simulink model "SHELL"  (Simulink 10.2)
settings: Solver=VariableStepAuto  StartTime=0.0  StopTime="sim_par.t_end  "  FixedStep=sim_par.dt  MaxStep="sim_par.t_step  "  RelTol="sim_par.rel_solver_tol "  EnableMultiTasking=on
libraries: OBSW x1, RWSW x1
settings Model: Creator=alger  LastModifiedBy=dbell44
settings DataIOCC: LimitDataPoints=on  SignalLoggingSaveFormat=Dataset
settings DebuggingCC: SolverPrmCheckMsg=warning  FcnCallInpInsideContextMsg=error  SignalLabelMismatchMsg=warning  UnconnectedLineMsg=error  RootOutportRequireBusObject=none  StateNameClashWarn=warning  StrictBusMsg=WarnOnBusTreatedAsVector  NonBusSignalsTreatedAsBus=warning
settings GRTTargetCC: CombineOutputUpdateFcns=on  GRTInterface=off

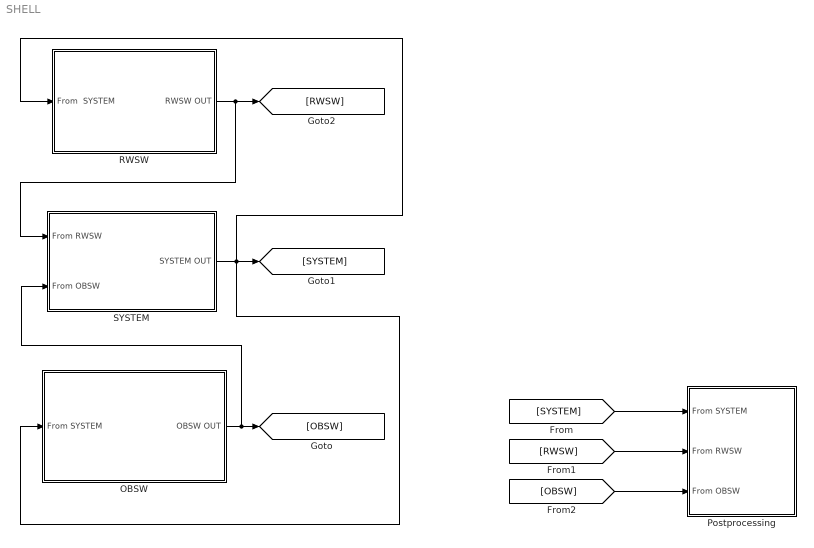
== system SHELL ==
  OBSW : Subsystem
  Postprocessing : Subsystem
  RWSW : Subsystem
  SYSTEM : Subsystem
  wires:
  OBSW/1(OBSW OUT) -> SYSTEM/2(From OBSW), [OBSW]
  [SYSTEM] -> Postprocessing/1(From SYSTEM)
  [RWSW] -> Postprocessing/2(From RWSW)
  [OBSW] -> Postprocessing/3("From OBSW ")
  RWSW/1(RWSW OUT) -> [RWSW], SYSTEM/1(From RWSW)
  SYSTEM/1("SYSTEM OUT ") -> [SYSTEM], OBSW/1(From SYSTEM), RWSW/1(From  SYSTEM)

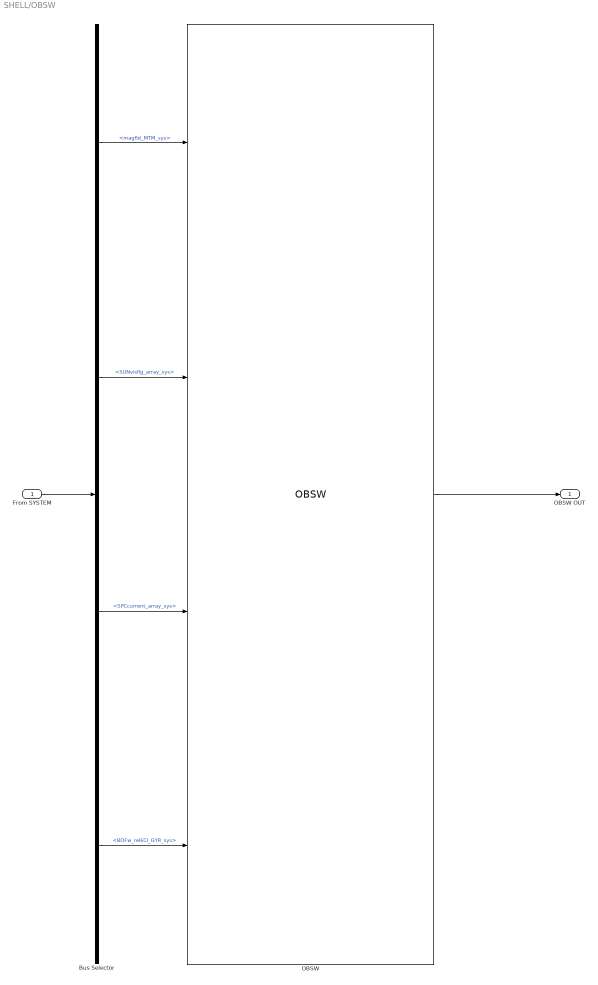
== system SHELL/OBSW ==
  From SYSTEM : Inport
  Bus Selector : BusSelector  OutputSignals=SYSSEN.magfld_MTM_sys,SYSSEN.SUNvisflg_array_sys,SYSSEN.SPCcurrent_array_sys,SYSSEN.BOFw_relECI_GYR_sys
  OBSW : OBSW/OBSW  SystemSampleTime=-1  VariantActivationTime=update diagram  Latency=0  AutoFrameSizeCalculation=off
  OBSW OUT : Outport
  wires:
  OBSW/1 -> OBSW OUT/1
  From SYSTEM/1 -> Bus Selector/1
  Bus Selector/1 -> OBSW/1  "<magfld_MTM_sys>"
  Bus Selector/2 -> OBSW/2  "<SUNvisflg_array_sys>"
  Bus Selector/3 -> OBSW/3  "<SPCcurrent_array_sys>"
  Bus Selector/4 -> OBSW/4  "<BOFw_relECI_GYR_sys>"

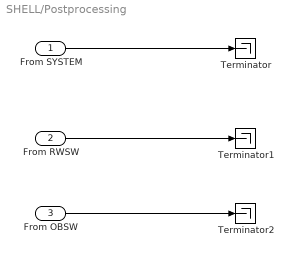
== system SHELL/Postprocessing ==
  From SYSTEM : Inport
  From RWSW : Inport  Port=2
  "From OBSW " : Inport  Port=3
  Terminator : Terminator
  Terminator1 : Terminator
  Terminator2 : Terminator
  wires:
  From SYSTEM/1 -> Terminator/1
  From RWSW/1 -> Terminator1/1
  "From OBSW "/1 -> Terminator2/1

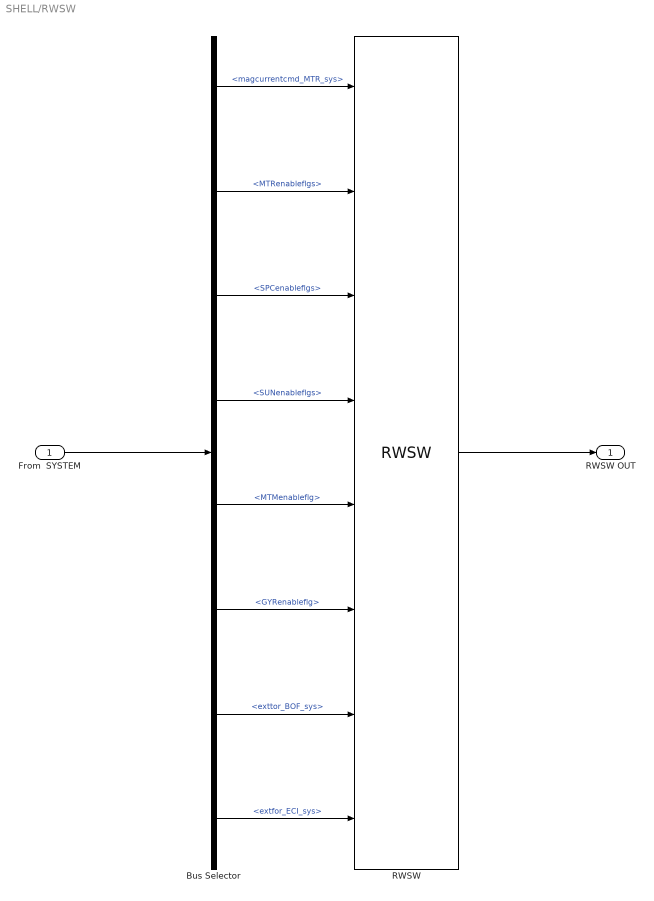
== system SHELL/RWSW ==
  From  SYSTEM : Inport
  Bus Selector : BusSelector  OutputSignals=SYSACT.magcurrentcmd_MTR_sys,SYSCMD.MTRenableflgs,SYSCMD.SPCenableflgs,SYSCMD.SUNenableflgs,SYSCMD.MTMenableflg,SYSCMD.GYRenableflg,SYSCMD.exttor_BOF_sys,SYSCMD.extfor_ECI_sys
  RWSW : RWSW/RWSW  SystemSampleTime=-1  VariantActivationTime=update diagram  Latency=0  AutoFrameSizeCalculation=off
  RWSW OUT : Outport
  wires:
  From  SYSTEM/1 -> Bus Selector/1
  Bus Selector/2 -> RWSW/2  "<MTRenableflgs>"
  Bus Selector/1 -> RWSW/1  "<magcurrentcmd_MTR_sys>"
  Bus Selector/5 -> RWSW/5  "<MTMenableflg>"
  Bus Selector/3 -> RWSW/3  "<SPCenableflgs>"
  Bus Selector/6 -> RWSW/6  "<GYRenableflg>"
  Bus Selector/4 -> RWSW/4  "<SUNenableflgs>"
  Bus Selector/7 -> RWSW/7  "<exttor_BOF_sys>"
  Bus Selector/8 -> RWSW/8  "<extfor_ECI_sys>"
  RWSW/1 -> RWSW OUT/1

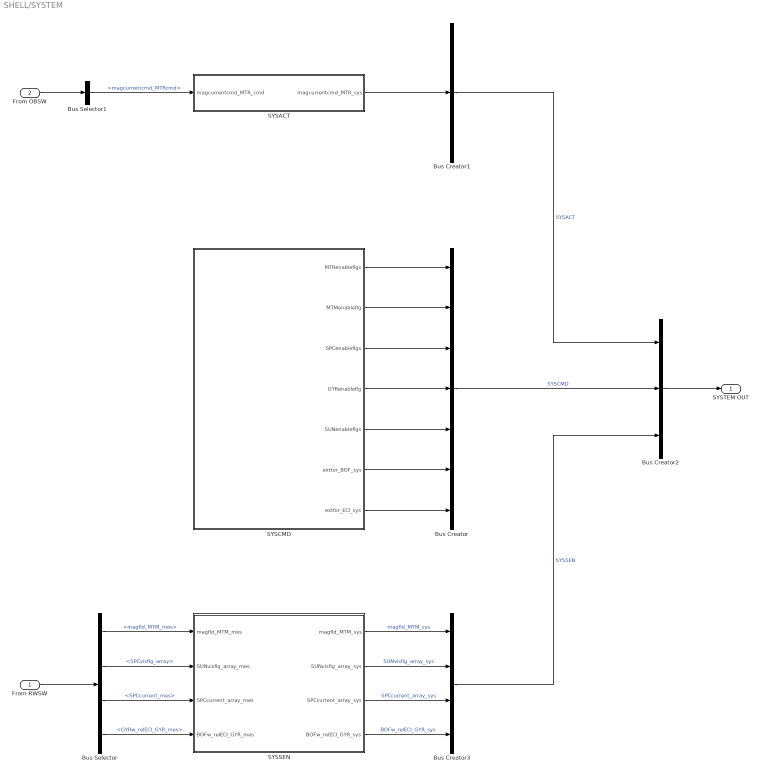
== system SHELL/SYSTEM ==
  From RWSW : Inport
  From OBSW : Inport  Port=2
  Bus Creator : BusCreator  Inputs=7
  Bus Creator1 : BusCreator  Inputs=1
  Bus Creator2 : BusCreator  Inputs=3
  Bus Creator3 : BusCreator  Inputs=4
  Bus Selector : BusSelector  OutputSignals=SEN.SEN_MTM.magfld_MTM_mes,SEN.SEN_SPC.SPCvisflg_array,SEN.SEN_SPC.SPCcurrent_mes,SEN.SEN_GYR.GYRw_relECI_GYR_mes
  Bus Selector1 : BusSelector  OutputSignals=magcurrentcmd_MTRcmd
  SYSACT : Subsystem
  SYSCMD : Subsystem
  SYSSEN : Subsystem
  "SYSTEM OUT " : Outport
  wires:
  From RWSW/1 -> Bus Selector/1
  Bus Creator/1 -> Bus Creator2/2  "SYSCMD"
  From OBSW/1 -> Bus Selector1/1
  SYSCMD/1(MTRenableflgs) -> Bus Creator/1
  SYSCMD/2(MTMenableflg) -> Bus Creator/2
  SYSCMD/3(SPCenableflgs) -> Bus Creator/3
  SYSCMD/4(GYRenableflg) -> Bus Creator/4
  SYSCMD/5(SUNenableflgs) -> Bus Creator/5
  SYSCMD/6(exttor_BOF_sys) -> Bus Creator/6
  SYSCMD/7(extfor_ECI_sys) -> Bus Creator/7
  Bus Creator1/1 -> Bus Creator2/1  "SYSACT"
  Bus Creator2/1 -> "SYSTEM OUT "/1
  Bus Creator3/1 -> Bus Creator2/3  "SYSSEN"
  Bus Selector/2 -> SYSSEN/2(SUNvisflg_array_mes)  "<SPCvisflg_array>"
  Bus Selector/3 -> SYSSEN/3(SPCcurrent_array_mes)  "<SPCcurrent_mes>"
  Bus Selector/1 -> SYSSEN/1(magfld_MTM_mes)  "<magfld_MTM_mes>"
  Bus Selector/4 -> SYSSEN/4(BOFw_relECI_GYR_mes)  "<GYRw_relECI_GYR_mes>"
  SYSSEN/1(magfld_MTM_sys) -> Bus Creator3/1  "magfld_MTM_sys"
  SYSSEN/2(SUNvisflg_array_sys) -> Bus Creator3/2  "SUNvisflg_array_sys"
  SYSSEN/3(SPCcurrent_array_sys) -> Bus Creator3/3  "SPCcurrent_array_sys"
  SYSSEN/4(BOFw_relECI_GYR_sys) -> Bus Creator3/4  "BOFw_relECI_GYR_sys"
  SYSACT/1(magcurrentcmd_MTR_sys) -> Bus Creator1/1
  Bus Selector1/1 -> SYSACT/1(magcurrentcmd_MTR_cmd)  "<magcurrentcmd_MTRcmd>"

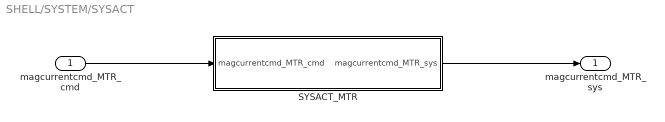
== system SHELL/SYSTEM/SYSACT ==
  magcurrentcmd_MTR_cmd : Inport
  SYSACT_MTR : Subsystem
  magcurrentcmd_MTR_sys : Outport
  wires:
  magcurrentcmd_MTR_cmd/1 -> SYSACT_MTR/1(magcurrentcmd_MTR_cmd)
  SYSACT_MTR/1(magcurrentcmd_MTR_sys) -> magcurrentcmd_MTR_sys/1

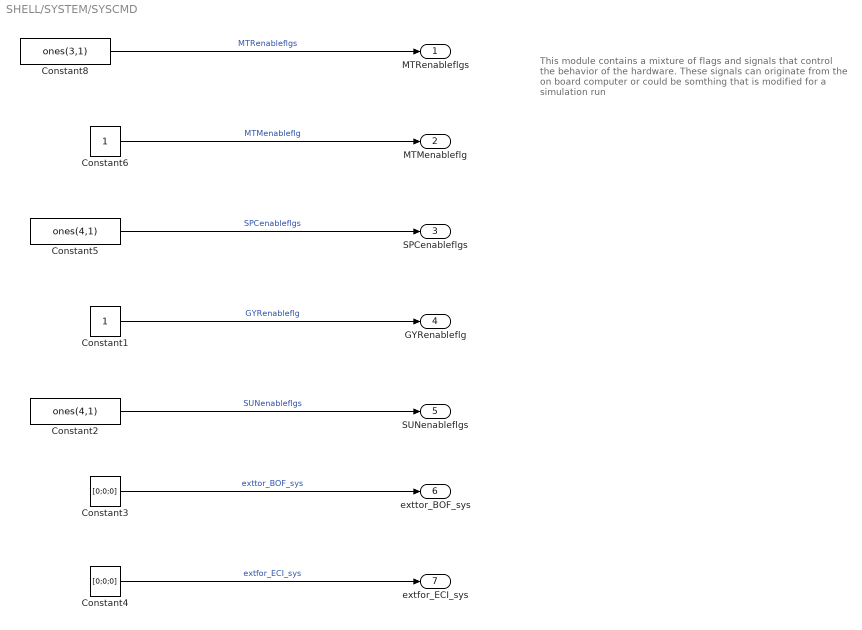
== system SHELL/SYSTEM/SYSCMD ==
  note: This module contains a mixture of  flags and signals that control the behavior of the
      | hardware.
      |
      | These signals can originate from the on board computer or could be somthing that is modified  for a simulation run
  Constant1 : Constant
  Constant2 : Constant  Value=ones(4,1)
  Constant3 : Constant  Value=[0;0;0]
  Constant4 : Constant  Value=[0;0;0]
  Constant5 : Constant  Value=ones(4,1)
  Constant6 : Constant
  Constant8 : Constant  Value=ones(3,1)
  MTRenableflgs : Outport
  MTMenableflg : Outport  Port=2
  SPCenableflgs : Outport  Port=3
  GYRenableflg : Outport  Port=4
  SUNenableflgs : Outport  Port=5
  exttor_BOF_sys : Outport  Port=6
  extfor_ECI_sys : Outport  Port=7
  wires:
  Constant3/1 -> exttor_BOF_sys/1  "exttor_BOF_sys"
  Constant8/1 -> MTRenableflgs/1  "MTRenableflgs"
  Constant2/1 -> SUNenableflgs/1  "SUNenableflgs"
  Constant6/1 -> MTMenableflg/1  "MTMenableflg"
  Constant1/1 -> GYRenableflg/1  "GYRenableflg"
  Constant4/1 -> extfor_ECI_sys/1  "extfor_ECI_sys"
  Constant5/1 -> SPCenableflgs/1  "SPCenableflgs"

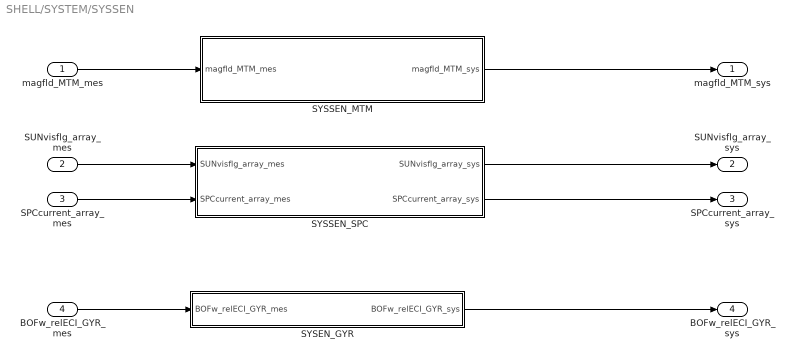
== system SHELL/SYSTEM/SYSSEN ==
  magfld_MTM_mes : Inport
  SUNvisflg_array_mes : Inport  Port=2
  SPCcurrent_array_mes : Inport  Port=3
  BOFw_relECI_GYR_mes : Inport  Port=4
  SYSEN_GYR : Subsystem
  SYSSEN_MTM : Subsystem
  SYSSEN_SPC : Subsystem
  magfld_MTM_sys : Outport
  SUNvisflg_array_sys : Outport  Port=2
  SPCcurrent_array_sys : Outport  Port=3
  BOFw_relECI_GYR_sys : Outport  Port=4
  wires:
  SPCcurrent_array_mes/1 -> SYSSEN_SPC/2(SPCcurrent_array_mes)
  SYSSEN_SPC/2(SPCcurrent_array_sys) -> SPCcurrent_array_sys/1
  SUNvisflg_array_mes/1 -> SYSSEN_SPC/1(SUNvisflg_array_mes)
  SYSSEN_SPC/1(SUNvisflg_array_sys) -> SUNvisflg_array_sys/1
  SYSSEN_MTM/1(magfld_MTM_sys) -> magfld_MTM_sys/1
  magfld_MTM_mes/1 -> SYSSEN_MTM/1(magfld_MTM_mes)
  BOFw_relECI_GYR_mes/1 -> SYSEN_GYR/1(BOFw_relECI_GYR_mes)
  SYSEN_GYR/1(BOFw_relECI_GYR_sys) -> BOFw_relECI_GYR_sys/1

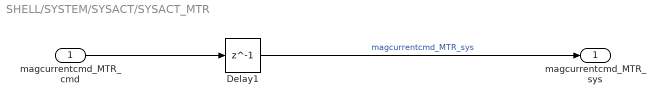
== system SHELL/SYSTEM/SYSACT/SYSACT_MTR ==
  magcurrentcmd_MTR_cmd : Inport
  Delay1 : Delay  DelayLength=1
  magcurrentcmd_MTR_sys : Outport
  wires:
  magcurrentcmd_MTR_cmd/1 -> Delay1/1
  Delay1/1 -> magcurrentcmd_MTR_sys/1  "magcurrentcmd_MTR_sys"

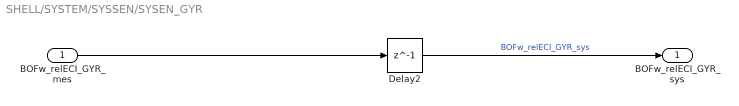
== system SHELL/SYSTEM/SYSSEN/SYSEN_GYR ==
  BOFw_relECI_GYR_mes : Inport
  Delay2 : Delay  DelayLength=1
  BOFw_relECI_GYR_sys : Outport
  wires:
  BOFw_relECI_GYR_mes/1 -> Delay2/1
  Delay2/1 -> BOFw_relECI_GYR_sys/1  "BOFw_relECI_GYR_sys"

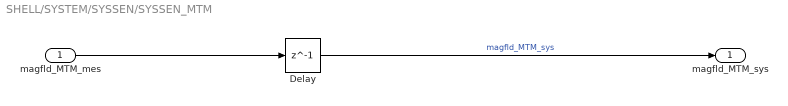
== system SHELL/SYSTEM/SYSSEN/SYSSEN_MTM ==
  magfld_MTM_mes : Inport
  Delay : Delay  DelayLength=1
  magfld_MTM_sys : Outport
  wires:
  magfld_MTM_mes/1 -> Delay/1
  Delay/1 -> magfld_MTM_sys/1  "magfld_MTM_sys"

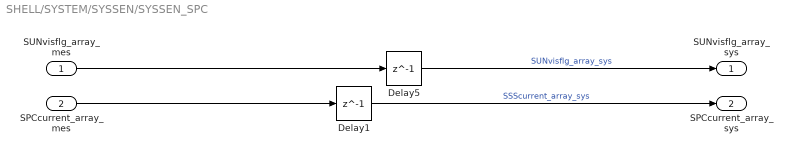
== system SHELL/SYSTEM/SYSSEN/SYSSEN_SPC ==
  SUNvisflg_array_mes : Inport
  SPCcurrent_array_mes : Inport  Port=2
  Delay1 : Delay  DelayLength=1
  Delay5 : Delay  DelayLength=1
  SUNvisflg_array_sys : Outport
  SPCcurrent_array_sys : Outport  Port=2
  wires:
  SUNvisflg_array_mes/1 -> Delay5/1
  SPCcurrent_array_mes/1 -> Delay1/1
  Delay1/1 -> SPCcurrent_array_sys/1  "SSScurrent_array_sys"
  Delay5/1 -> SUNvisflg_array_sys/1  "SUNvisflg_array_sys"
